simulink model "Control_linear2012b"  (R2012b)
settings: Solver=ode3  SolverMode=SingleTasking  StartTime=0.0  StopTime=50  FixedStep=0.005  RelTol=1e-3
values from neighbouring files (symbols this model uses):
  a1 = 0.2634    [int_for_newsimu.m]
  a2 = 1.6279    [int_for_newsimu.m]
  a3 = 25.6488    [int_for_newsimu.m]
  b1 = 0.531    [int_for_newsimu.m]
  b2 = 5.3292    [int_for_newsimu.m]
  epsilon_d = epsilon    (= 0)    [int_for_newsimu.m]
  fd = a3*cos(epsilon)*sin(theta)/b2    [int_for_newsimu.m]
  K_psi2theta = [1.8,0.2]    [int_for_newsimu.m]
  n = 0.9    [int_for_newsimu.m]
  theta_d = theta    (= 0)    [int_for_newsimu.m]
  w = 100    [int_for_newsimu.m]
undefined symbols (not defined in the file or in its folder): K
libraries: dspsrcs4 x9
settings Model: SimulationMode=external  ExtModeTrigDuration=200000  Creator=5420  LastModifiedBy=yk.L
settings DataIOCC: SignalLoggingSaveFormat=ModelDataLogs  SignalLoggingName=sigsOut
settings OptimizationCC: InitFltsAndDblsToZero=on
settings DebuggingCC: SaveWithParameterizedLinksMsg=none  SignalResolutionControl=TryResolveAllWithWarning  SolverPrmCheckMsg=none  MultiTaskDSMMsg=warning  MultiTaskCondExecSysMsg=none  FrameProcessingCompatibilityMsg=error
settings HardwareCC: ProdBitPerPointer=64  ProdLargestAtomicFloat=Float  ProdIntDivRoundTo=Zero  ProdEndianess=LittleEndian  ProdHWDeviceType=Specified
settings RTWCC: SystemTargetFile=rtwin.tlc  TemplateMakefile=rtwin.tmf  Description=Simulink Desktop Real-Time  ProcessScript=rtwin_make_rtw_hook  RTWCompilerOptimization=On
settings CodeAppCC: MaxIdLength=95
settings RTWinTargetCC: TargetPreCompLibLocation=D:\Program Files (x86)\MatlabR21019b\toolbox\sldrt\lib\win64  CodeReplacementLibrary=C89/C90 (ANSI)  ModelReferenceCompliant=off  CompOptLevelCompliant=off  RTWinDir=C:/PROGRA~1/MATLAB/R2012b/toolbox/rtw/targets/rtwin  TargetArch=win32  ExtModeMexFile=sldrtext

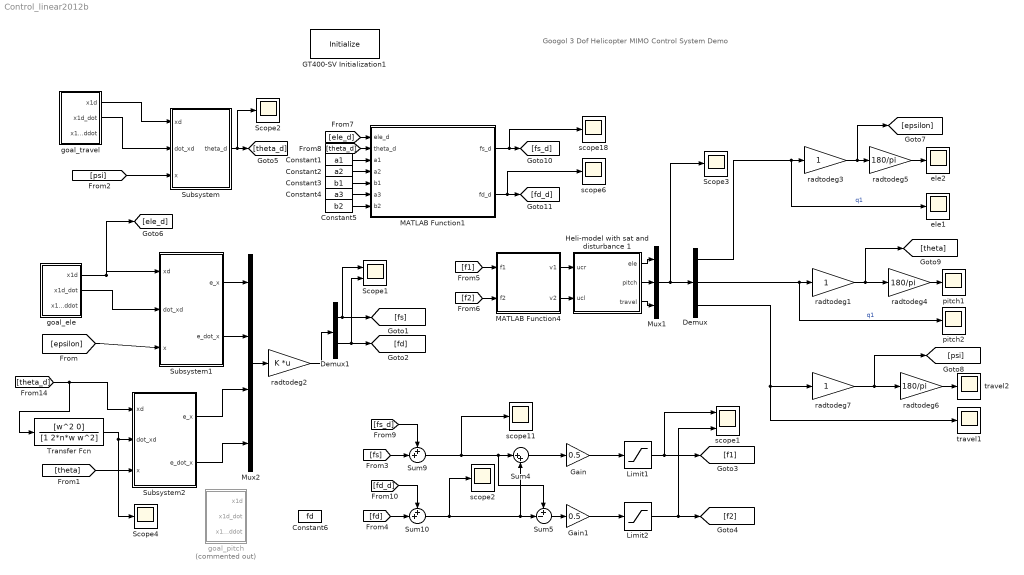
== system Control_linear2012b ==
  note: Googol 3 Dof Helicopter MIMO Control System Demo
  Constant1 : Constant  Value=a1
  Constant2 : Constant  Value=a2
  Constant3 : Constant  Value=b1
  Constant4 : Constant  Value=a3
  Constant5 : Constant  Value=b2
  Constant6 : Constant  Value=fd
  Demux : Demux  Outputs=3
  Demux1 : Demux  Outputs=2
  GT400-SV Initialization1 : S-Function  Priority=0  FunctionName=Initialize  Parameters=openloop  EnableBusSupport=off  mask(Initialize){openloop=1}
      mask prompts: openloop "Control loop:"
      mask help:
      | Initializing the googol GT400-SV motion control board.
      | Block parameter:
      |     Control loop:
      |          0: closed-loop control.
      |          1: opened-loop control.
      mask Help: This initialize block initializes the googol GT400-SV motion control board.
      mask Display: disp('Initialize \nGT400-SV');
  Gain : Gain  Gain=0.5
  Gain1 : Gain  Gain=0.5
  Heli-model with sat and disturbance 1 : Subsystem
  Limit1 : Saturate  UpperLimit=4  LowerLimit=0.05
  Limit2 : Saturate  UpperLimit=4  LowerLimit=0.05
  MATLAB Function1 : MATLAB Function  TreatAsAtomicUnit=on
  MATLAB Function4 : MATLAB Function  TreatAsAtomicUnit=on
  Mux1 : Mux  Inputs=3
  Mux2 : Mux
  Scope1 : Scope  NumInputPorts=2
      settings: YMin=-142.35203~-10.42115  YMax=297.12256~15.56883
  Scope2 : Scope
      settings: YMin=-0.02728  YMax=0.19696  SaveName=ScopeData2
  Scope3 : Scope
      settings: YMin=-1.59949  YMax=8.94541  SaveName=ScopeData18
  Scope4 : Scope
      settings: YMin=-0.02728  YMax=0.19696  SaveName=ScopeData6
  Subsystem : Subsystem
  Subsystem1 : Subsystem
  Subsystem2 : Subsystem
  Sum10 : Sum  Inputs=++|
  Sum4 : Sum  Inputs=|++
  Sum5 : Sum  Inputs=+-|
  Sum9 : Sum  Inputs=++|
  Transfer Fcn : TransferFcn  Numerator=[w^2 0]  Denominator=[1 2*n*w w^2]
  ele1 : Scope
      settings: YMin=-1.23857  YMax=0.24711  SaveName=elevation_real_data
  ele2 : Scope
      settings: YMin=4.45  YMax=4.775  SaveName=elevation_real_data1
  goal_ele : Subsystem
  goal_pitch : Subsystem  Commented=on
  goal_travel : Subsystem
  pitch1 : Scope
      settings: YMin=-12.5  YMax=-1  SaveName=pitch_real_data1
  pitch2 : Scope
      settings: YMin=-12.5  YMax=-1  SaveName=pitch_real_data
  radtodeg1 : Gain
  radtodeg2 : Gain  Gain=K  Multiplication=Matrix(K*u)
  radtodeg3 : Gain
  radtodeg4 : Gain  Gain=180/pi
  radtodeg5 : Gain  Gain=180/pi
  radtodeg6 : Gain  Gain=180/pi
  radtodeg7 : Gain
  scope1 : Scope  NumInputPorts=2
      settings: YMin=-0.44375~-0.44375  YMax=4.49375~4.49375  SaveName=ScopeData11
  scope{2,6,11,18} (4 alike) : Scope
      scope11 settings: YMin=-2.5  YMax=7.5  SaveName=fs_data
      scope18 settings: YMin=3.015  YMax=3.10151  SaveName=fs_d
      scope2 settings: YMin=-2.5  YMax=7.5  SaveName=fd_data
      scope6 settings: YMin=-0.2097  YMax=0.2097  SaveName=fd_d
  travel1 : Scope
      settings: YMin=295  YMax=327.5  SaveName=tralvel_real_data
  travel2 : Scope
      settings: YMin=295  YMax=327.5  SaveName=tralvel_real_data1
  wires:
  radtodeg5/1 -> ele2/1
  Demux/2 -> pitch2/1, radtodeg1/1  "q1"
  radtodeg6/1 -> travel2/1
  Demux/3 -> travel1/1, radtodeg7/1
  Mux1/1 -> Scope3/1, Demux/1
  Heli-model with sat and disturbance 1/1(ele) -> Mux1/1
  Heli-model with sat and disturbance 1/2(pitch) -> Mux1/2
  Heli-model with sat and disturbance 1/3(travel) -> Mux1/3
  Demux/1 -> ele1/1, radtodeg3/1  "q1"
  radtodeg4/1 -> pitch1/1
  Mux2/1 -> radtodeg2/1
  radtodeg2/1 -> Demux1/1
  Sum10/1 -> scope2/1, Sum5/2, Sum4/2
  Sum4/1 -> Gain/1
  Sum9/1 -> scope11/1, Sum5/1, Sum4/1
  Sum5/1 -> Gain1/1
  Gain/1 -> Limit1/1
  Gain1/1 -> Limit2/1
  Limit1/1 -> scope1/1, [f1]
  Limit2/1 -> [f2], scope1/2
  Demux1/1 -> Scope1/1, [fs]
  Demux1/2 -> Scope1/2, [fd]
  [f1] -> MATLAB Function4/1(f1)
  [f2] -> MATLAB Function4/2(f2)
  radtodeg1/1 -> [theta], radtodeg4/1
  radtodeg3/1 -> [epsilon], radtodeg5/1
  radtodeg7/1 -> radtodeg6/1, [psi]
  [theta_d] -> Transfer Fcn/1, Subsystem2/1(xd)
  [fs] -> Sum9/2
  [fd] -> Sum10/2
  [ele_d] -> MATLAB Function1/1(ele_d)
  [theta_d] -> MATLAB Function1/2(theta_d)
  Constant1/1 -> MATLAB Function1/3(a1)
  Constant2/1 -> MATLAB Function1/4(a2)
  Constant3/1 -> MATLAB Function1/5(b1)
  Constant4/1 -> MATLAB Function1/6(a3)
  Constant5/1 -> MATLAB Function1/7(b2)
  MATLAB Function1/1(fs_d) -> scope18/1, [fs_d]
  MATLAB Function1/2(fd_d) -> scope6/1, [fd_d]
  goal_travel/1(x1d) -> Subsystem/1(xd)
  goal_travel/2(x1d_dot) -> Subsystem/2(dot_xd)
  [psi] -> Subsystem/3(x)
  goal_ele/1(x1d) -> [ele_d], Subsystem1/1(xd)
  goal_ele/2(x1d_dot) -> Subsystem1/2(dot_xd)
  [epsilon] -> Subsystem1/3(x)
  Transfer Fcn/1 -> Subsystem2/2(dot_xd), Scope4/1
  [theta] -> Subsystem2/3(x)
  [fs_d] -> Sum9/1
  [fd_d] -> Sum10/1
  Subsystem1/1(e_x) -> Mux2/1
  Subsystem1/2(e_dot_x) -> Mux2/2
  Subsystem2/1(e_x) -> Mux2/3
  Subsystem2/2(e_dot_x) -> Mux2/4
  Subsystem/1(theta_d) -> Scope2/1, [theta_d]
  MATLAB Function4/1(v1) -> Heli-model with sat and disturbance 1/1(ucr)
  MATLAB Function4/2(v2) -> Heli-model with sat and disturbance 1/2(ucl)

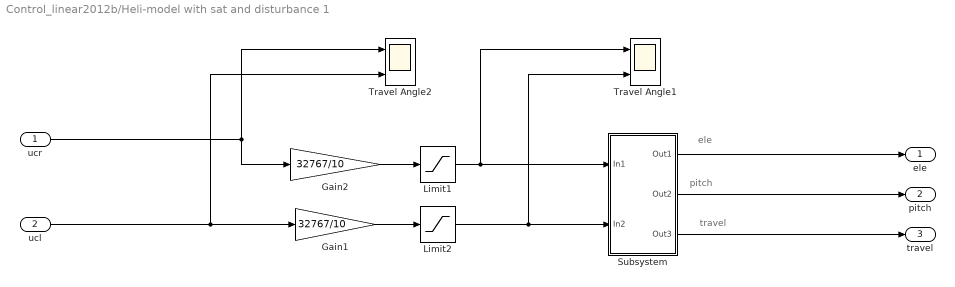
== system Control_linear2012b/Heli-model with sat and disturbance 1 ==
  note: travel
  note: pitch
  note: ele
  ucr : Inport
  ucl : Inport  Port=2
  Gain1 : Gain  Gain=32767/10
  Gain2 : Gain  Gain=32767/10
  Limit1 : Saturate  UpperLimit=15000  LowerLimit=-15000
  Limit2 : Saturate  UpperLimit=15000  LowerLimit=-15000
  Subsystem : Subsystem
  Travel Angle1 : Scope  NumInputPorts=2
      settings: TimeRange=200  YMin=0~0  YMax=3500~3500  SaveName=travel1  MaxDataPoints=200000
  Travel Angle2 : Scope  NumInputPorts=2
      settings: TimeRange=200  YMin=0.3~0.3  YMax=0.7~0.7  SaveName=travel  MaxDataPoints=200000
  ele : Outport
  pitch : Outport  Port=2
  travel : Outport  Port=3
  wires:
  Subsystem/1(Out1) -> ele/1
  Subsystem/2(Out2) -> pitch/1
  Subsystem/3(Out3) -> travel/1
  Gain2/1 -> Limit1/1
  Gain1/1 -> Limit2/1
  Limit1/1 -> Travel Angle1/1, Subsystem/1(In1)
  Limit2/1 -> Travel Angle1/2, Subsystem/2(In2)
  ucr/1 -> Gain2/1, Travel Angle2/1
  ucl/1 -> Travel Angle2/2, Gain1/1

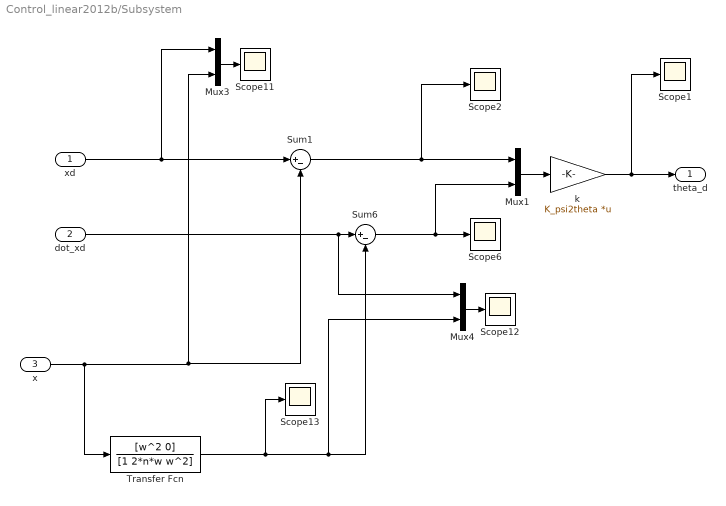
== system Control_linear2012b/Subsystem ==
  xd : Inport
  dot_xd : Inport  Port=2
  x : Inport  Port=3
  Mux1 : Mux  Inputs=2
  Mux3 : Mux  Inputs=2
  Mux4 : Mux  Inputs=2
  Scope{1..2,6,11..13} (6 alike) : Scope
      Scope1 settings: YMin=-0.02728  YMax=0.19696
      Scope11 settings: TimeRange=50  YMin=-0.02184  YMax=0.19654  SaveName=ScopeData3
      Scope12 settings: YMin=-0.49275  YMax=-0.4885  SaveName=ScopeData16
      Scope13 settings: YMin=0.0013  YMax=0.0027  SaveName=ScopeData17
      Scope2 settings: YMin=-0.02201  YMax=0.19637  SaveName=ScopeData19
      Scope6 settings: YMin=-0.0879  YMax=0.00986  SaveName=ScopeData20
  Sum1 : Sum  Inputs=|+-
  Sum6 : Sum  Inputs=|+-
  Transfer Fcn : TransferFcn  Numerator=[w^2 0]  Denominator=[1 2*n*w w^2]
  k : Gain  Gain=K_psi2theta  Multiplication=Matrix(K*u)
  theta_d : Outport
  wires:
  dot_xd/1 -> Mux4/1, Sum6/1
  x/1 -> Transfer Fcn/1, Sum1/2, Mux3/2
  Transfer Fcn/1 -> Scope13/1, Mux4/2, Sum6/2
  Sum6/1 -> Mux1/2, Scope6/1
  Mux3/1 -> Scope11/1
  Mux4/1 -> Scope12/1
  Sum1/1 -> Mux1/1, Scope2/1
  xd/1 -> Mux3/1, Sum1/1
  Mux1/1 -> k/1
  k/1 -> Scope1/1, theta_d/1

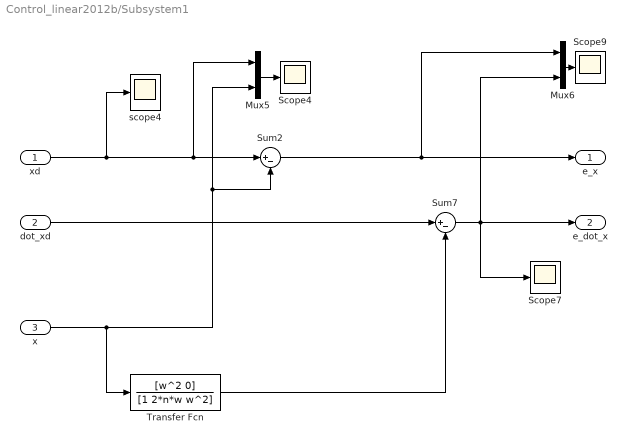
== system Control_linear2012b/Subsystem1 ==
  xd : Inport
  dot_xd : Inport  Port=2
  x : Inport  Port=3
  Mux5 : Mux  Inputs=2
  Mux6 : Mux  Inputs=2
  Scope4 : Scope
      settings: YMin=-0.61494  YMax=0.08442  SaveName=ScopeData4
  Scope7 : Scope
      settings: YMin=-1  YMax=12  SaveName=ScopeData7
  Scope9 : Scope
      settings: YMin=-0.52  YMax=-0.4875  SaveName=ScopeData12
  Sum2 : Sum  Inputs=|+-
  Sum7 : Sum  Inputs=|+-
  Transfer Fcn : TransferFcn  Numerator=[w^2 0]  Denominator=[1 2*n*w w^2]
  scope4 : Scope
      settings: YMin=-2.5  YMax=7.5  SaveName=ele_d_data  DataFormat=Structure
  e_x : Outport
  e_dot_x : Outport  Port=2
  wires:
  xd/1 -> Mux5/1, Sum2/1, scope4/1
  Mux6/1 -> Scope9/1
  Mux5/1 -> Scope4/1
  Transfer Fcn/1 -> Sum7/2
  x/1 -> Transfer Fcn/1, Mux5/2, Sum2/2
  Sum7/1 -> Mux6/2, e_dot_x/1, Scope7/1
  Sum2/1 -> e_x/1, Mux6/1
  dot_xd/1 -> Sum7/1

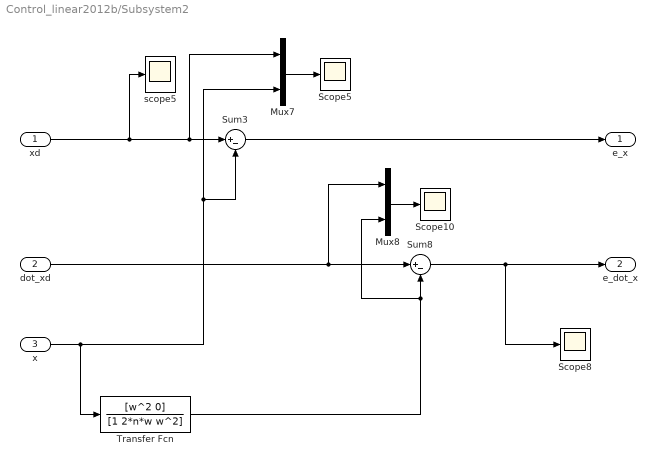
== system Control_linear2012b/Subsystem2 ==
  xd : Inport
  dot_xd : Inport  Port=2
  x : Inport  Port=3
  Mux7 : Mux  Inputs=2
  Mux8 : Mux  Inputs=2
  Scope10 : Scope
      settings: YMin=-0.08392  YMax=0.52488  SaveName=ScopeData13
  Scope5 : Scope
      settings: YMin=-0.02741  YMax=0.19697  SaveName=ScopeData5
  Scope8 : Scope
      settings: YMin=-1  YMax=12  SaveName=ScopeData10
  Sum3 : Sum  Inputs=|+-
  Sum8 : Sum  Inputs=|+-
  Transfer Fcn : TransferFcn  Numerator=[w^2 0]  Denominator=[1 2*n*w w^2]
  scope5 : Scope
      settings: YMin=-2.5  YMax=7.5  SaveName=pitch_d_data  DataFormat=Structure
  e_x : Outport
  e_dot_x : Outport  Port=2
  wires:
  Sum3/1 -> e_x/1
  Transfer Fcn/1 -> Sum8/2, Mux8/2
  Sum8/1 -> Scope8/1, e_dot_x/1
  xd/1 -> scope5/1, Mux7/1, Sum3/1
  x/1 -> Transfer Fcn/1, Sum3/2, Mux7/2
  Mux8/1 -> Scope10/1
  dot_xd/1 -> Sum8/1, Mux8/1
  Mux7/1 -> Scope5/1

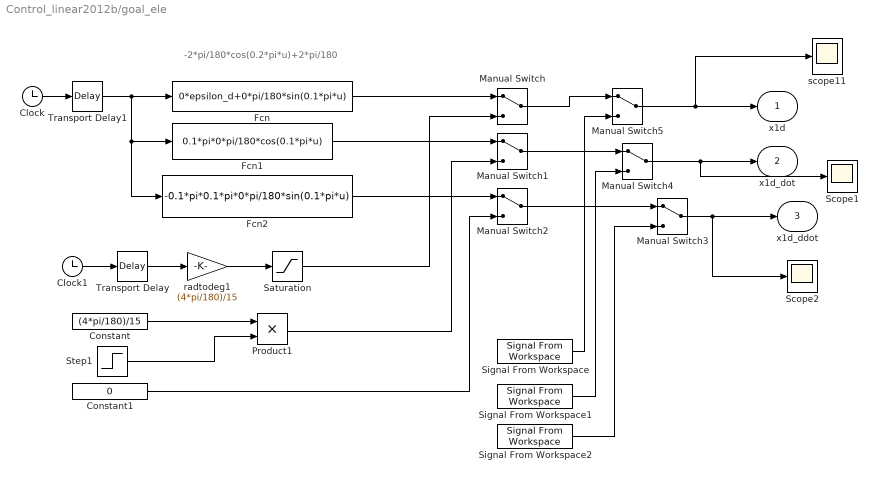
== system Control_linear2012b/goal_ele ==
  note: -2*pi/180*cos(0.2*pi*u)+2*pi/180
  Clock : Clock
  Clock1 : Clock
  Constant : Constant  Value=(4*pi/180)/15
  Constant1 : Constant  Value=0
  Fcn : Fcn  Expr=0*epsilon_d+0*pi/180*sin(0.1*pi*u)
  Fcn1 : Fcn  Expr=0.1*pi*0*pi/180*cos(0.1*pi*u)
  Fcn2 : Fcn  Expr=-0.1*pi*0.1*pi*0*pi/180*sin(0.1*pi*u)
  Manual Switch{,1..5} (6 alike) : ManualSwitch
  Product1 : Product  RndMeth=Zero
  Saturation : Saturate  UpperLimit=(4*pi/180)  LowerLimit=-(4*pi/180)
  Scope1 : Scope
      settings: YMin=-10  YMax=10  SaveName=ScopeData8
  Scope2 : Scope
      settings: YMin=-10  YMax=10  SaveName=ScopeData9
  Signal From Workspace : dspsrcs4/Signal From Workspace  X=epsilon  Ts=0.005  nsamps=1  OutputAfterFinalValue=Setting to zero  ignoreOrWarnInputAndFrameLengths=off
  Signal From Workspace1 : dspsrcs4/Signal From Workspace  X=dot_epsilon  Ts=0.005  nsamps=1  OutputAfterFinalValue=Setting to zero  ignoreOrWarnInputAndFrameLengths=off
  Signal From Workspace2 : dspsrcs4/Signal From Workspace  X=ddot_epsilon  Ts=0.005  nsamps=1  OutputAfterFinalValue=Setting to zero  ignoreOrWarnInputAndFrameLengths=off
  Step1 : Step  Time=12  SampleTime=0
  Transport Delay : TransportDelay  DelayTime=12
  Transport Delay1 : TransportDelay  DelayTime=0
  radtodeg1 : Gain  Gain=(4*pi/180)/15
  scope11 : Scope
      settings: YMin=-2.5  YMax=7.5  SaveName=ele_d_data
  x1d : Outport
  x1d_dot : Outport  Port=2
  x1d_ddot : Outport  Port=3
  wires:
  Clock/1 -> Transport Delay1/1
  Clock1/1 -> Transport Delay/1
  Transport Delay/1 -> radtodeg1/1
  radtodeg1/1 -> Saturation/1
  Fcn/1 -> Manual Switch/1
  Fcn1/1 -> Manual Switch1/1
  Fcn2/1 -> Manual Switch2/1
  Manual Switch2/1 -> Manual Switch3/1
  Saturation/1 -> Manual Switch/2
  Constant1/1 -> Manual Switch2/2
  Constant/1 -> Product1/1
  Step1/1 -> Product1/2
  Product1/1 -> Manual Switch1/2
  Transport Delay1/1 -> Fcn1/1, Fcn2/1, Fcn/1
  Signal From Workspace2/1 -> Manual Switch3/2
  Manual Switch3/1 -> Scope2/1, x1d_ddot/1
  Signal From Workspace1/1 -> Manual Switch4/2
  Manual Switch1/1 -> Manual Switch4/1
  Manual Switch4/1 -> Scope1/1, x1d_dot/1
  Manual Switch/1 -> Manual Switch5/1
  Signal From Workspace/1 -> Manual Switch5/2
  Manual Switch5/1 -> scope11/1, x1d/1

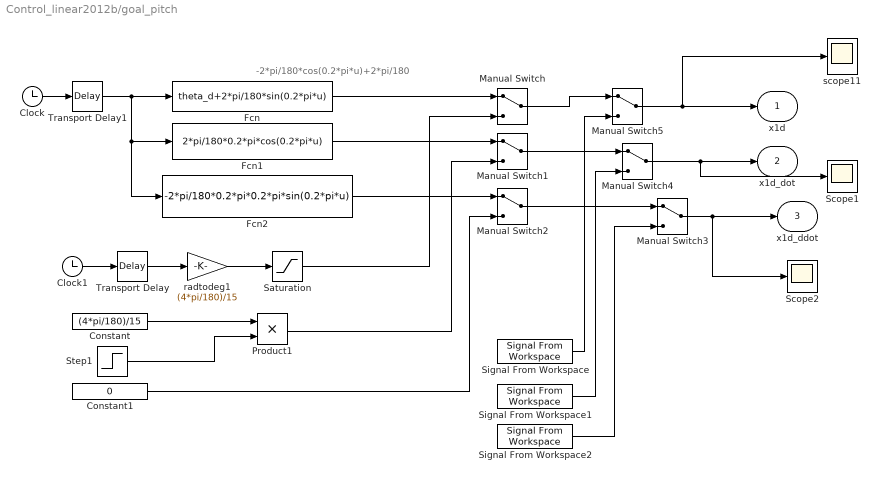
== system Control_linear2012b/goal_pitch ==
  note: -2*pi/180*cos(0.2*pi*u)+2*pi/180
  Clock : Clock
  Clock1 : Clock
  Constant : Constant  Value=(4*pi/180)/15
  Constant1 : Constant  Value=0
  Fcn : Fcn  Expr=theta_d+2*pi/180*sin(0.2*pi*u)
  Fcn1 : Fcn  Expr=2*pi/180*0.2*pi*cos(0.2*pi*u)
  Fcn2 : Fcn  Expr=-2*pi/180*0.2*pi*0.2*pi*sin(0.2*pi*u)
  Manual Switch{,1..5} (6 alike) : ManualSwitch
  Product1 : Product  RndMeth=Zero
  Saturation : Saturate  UpperLimit=(4*pi/180)  LowerLimit=-(4*pi/180)
  Scope1 : Scope
      settings: YMin=-10  YMax=10  SaveName=ScopeData8
  Scope2 : Scope
      settings: YMin=-10  YMax=10  SaveName=ScopeData9
  Signal From Workspace : dspsrcs4/Signal From Workspace  X=epsilon  Ts=0.005  nsamps=1  OutputAfterFinalValue=Setting to zero  ignoreOrWarnInputAndFrameLengths=off
  Signal From Workspace1 : dspsrcs4/Signal From Workspace  X=dot_epsilon  Ts=0.005  nsamps=1  OutputAfterFinalValue=Setting to zero  ignoreOrWarnInputAndFrameLengths=off
  Signal From Workspace2 : dspsrcs4/Signal From Workspace  X=ddot_epsilon  Ts=0.005  nsamps=1  OutputAfterFinalValue=Setting to zero  ignoreOrWarnInputAndFrameLengths=off
  Step1 : Step  Time=12  SampleTime=0
  Transport Delay : TransportDelay  DelayTime=12
  Transport Delay1 : TransportDelay  DelayTime=0
  radtodeg1 : Gain  Gain=(4*pi/180)/15
  scope11 : Scope
      settings: YMin=-2.5  YMax=7.5  SaveName=pitch_d_data
  x1d : Outport
  x1d_dot : Outport  Port=2
  x1d_ddot : Outport  Port=3
  wires:
  Clock/1 -> Transport Delay1/1
  Clock1/1 -> Transport Delay/1
  Transport Delay/1 -> radtodeg1/1
  radtodeg1/1 -> Saturation/1
  Fcn/1 -> Manual Switch/1
  Fcn1/1 -> Manual Switch1/1
  Fcn2/1 -> Manual Switch2/1
  Manual Switch2/1 -> Manual Switch3/1
  Saturation/1 -> Manual Switch/2
  Constant1/1 -> Manual Switch2/2
  Constant/1 -> Product1/1
  Step1/1 -> Product1/2
  Product1/1 -> Manual Switch1/2
  Transport Delay1/1 -> Fcn1/1, Fcn2/1, Fcn/1
  Signal From Workspace2/1 -> Manual Switch3/2
  Manual Switch3/1 -> Scope2/1, x1d_ddot/1
  Signal From Workspace1/1 -> Manual Switch4/2
  Manual Switch1/1 -> Manual Switch4/1
  Manual Switch4/1 -> Scope1/1, x1d_dot/1
  Manual Switch/1 -> Manual Switch5/1
  Signal From Workspace/1 -> Manual Switch5/2
  Manual Switch5/1 -> scope11/1, x1d/1

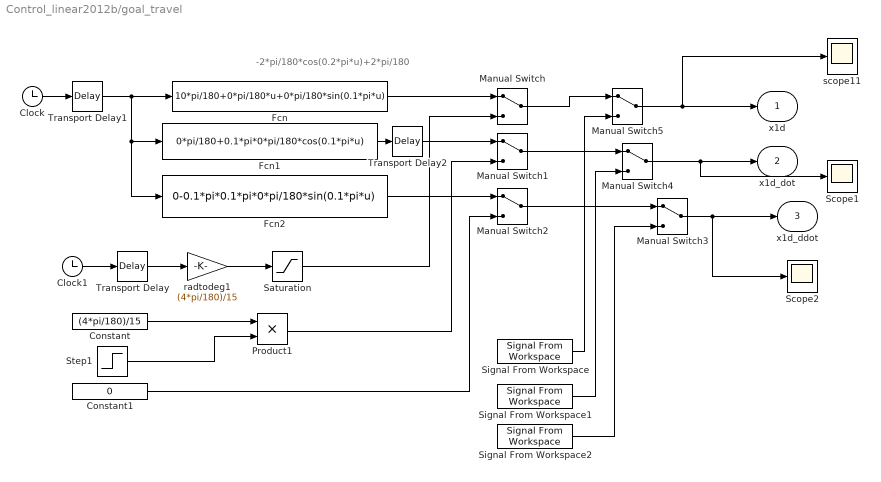
== system Control_linear2012b/goal_travel ==
  note: -2*pi/180*cos(0.2*pi*u)+2*pi/180
  Clock : Clock
  Clock1 : Clock
  Constant : Constant  Value=(4*pi/180)/15
  Constant1 : Constant  Value=0
  Fcn : Fcn  Expr=10*pi/180+0*pi/180*u+0*pi/180*sin(0.1*pi*u)
  Fcn1 : Fcn  Expr=0*pi/180+0.1*pi*0*pi/180*cos(0.1*pi*u)
  Fcn2 : Fcn  Expr=0-0.1*pi*0.1*pi*0*pi/180*sin(0.1*pi*u)
  Manual Switch{,1..5} (6 alike) : ManualSwitch
  Product1 : Product  RndMeth=Zero
  Saturation : Saturate  UpperLimit=(4*pi/180)  LowerLimit=-(4*pi/180)
  Scope1 : Scope
      settings: YMin=-0.01309  YMax=0.11781  SaveName=ScopeData8
  Scope2 : Scope
      settings: YMin=-1.00000  YMax=1.00000  SaveName=ScopeData9
  Signal From Workspace : dspsrcs4/Signal From Workspace  X=epsilon  Ts=0.005  nsamps=1  OutputAfterFinalValue=Setting to zero  ignoreOrWarnInputAndFrameLengths=off
  Signal From Workspace1 : dspsrcs4/Signal From Workspace  X=dot_epsilon  Ts=0.005  nsamps=1  OutputAfterFinalValue=Setting to zero  ignoreOrWarnInputAndFrameLengths=off
  Signal From Workspace2 : dspsrcs4/Signal From Workspace  X=ddot_epsilon  Ts=0.005  nsamps=1  OutputAfterFinalValue=Setting to zero  ignoreOrWarnInputAndFrameLengths=off
  Step1 : Step  Time=12  SampleTime=0
  Transport Delay : TransportDelay  DelayTime=12
  Transport Delay1 : TransportDelay  DelayTime=10
  Transport Delay2 : TransportDelay  DelayTime=10
  radtodeg1 : Gain  Gain=(4*pi/180)/15
  scope11 : Scope
      settings: YMin=-2.5  YMax=7.5  SaveName=travel_d_data
  x1d : Outport
  x1d_dot : Outport  Port=2
  x1d_ddot : Outport  Port=3
  wires:
  Clock/1 -> Transport Delay1/1
  Clock1/1 -> Transport Delay/1
  Transport Delay/1 -> radtodeg1/1
  radtodeg1/1 -> Saturation/1
  Manual Switch2/1 -> Manual Switch3/1
  Saturation/1 -> Manual Switch/2
  Constant1/1 -> Manual Switch2/2
  Constant/1 -> Product1/1
  Step1/1 -> Product1/2
  Product1/1 -> Manual Switch1/2
  Transport Delay1/1 -> Fcn1/1, Fcn2/1, Fcn/1
  Signal From Workspace2/1 -> Manual Switch3/2
  Manual Switch3/1 -> Scope2/1, x1d_ddot/1
  Signal From Workspace1/1 -> Manual Switch4/2
  Manual Switch1/1 -> Manual Switch4/1
  Manual Switch4/1 -> Scope1/1, x1d_dot/1
  Manual Switch/1 -> Manual Switch5/1
  Signal From Workspace/1 -> Manual Switch5/2
  Manual Switch5/1 -> scope11/1, x1d/1
  Fcn/1 -> Manual Switch/1
  Fcn1/1 -> Transport Delay2/1
  Fcn2/1 -> Manual Switch2/1
  Transport Delay2/1 -> Manual Switch1/1

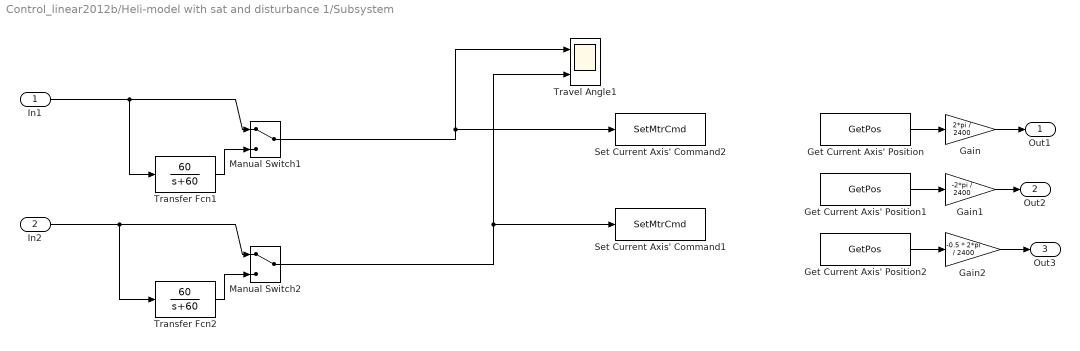
== system Control_linear2012b/Heli-model with sat and disturbance 1/Subsystem ==
  In1 : Inport
  In2 : Inport  Port=2
  Gain : Gain  Gain=2*pi / 2400  SaturateOnIntegerOverflow=on  OutDataTypeStr=Inherit: Same as input  ParamDataTypeStr=Inherit: Same as input
  Gain1 : Gain  Gain=-2*pi / 2400  SaturateOnIntegerOverflow=on  OutDataTypeStr=Inherit: Same as input  ParamDataTypeStr=Inherit: Same as input
  Gain2 : Gain  Gain=-0.5 * 2*pi / 2400  SaturateOnIntegerOverflow=on  OutDataTypeStr=Inherit: Same as input  ParamDataTypeStr=Inherit: Same as input
  Get Current Axis' Position : S-Function  Priority=1  FunctionName=GetPos  Parameters=axis  EnableBusSupport=off  mask(GetPos){axis=2}
      mask prompts: axis "Axis number:"
      mask help:
      | Getting the current axis position value in encoder' counts.
      | Block parameter:
      |     Axis number:  must be between 1 and 6, default is 1.
      | Block output:
      |     1~4: current axis' encoder reading counts.
      |     5/6: assistant encoder 1/2 reading counts.
      mask Help:
      | This block, GetPos, is intended for getting the current axis position value in encoder' counts. This value represents the actual position for the axis
      | at the current sample time. This command operates for all profile modes.
      | The value returned is a 32-bit signed number with units of counts.
      | The range is -1,073,741,824 to 1,073,741,823.
      | 
      | You can recalculate obtained value into meter units via multiplication by the scaler coefficient .
      | 
      | Block parameter:
      |     Axis number:  must be between 1 and 4, default is 1.
      | Block input: none.
      | Block output:
      |         1~4: current axis' encoder reading counts.
      |         5/6: assistant encoder 1/2 reading counts.
      mask Display:
      | disp('GetPos');
      | port_label('output', 1, 'Pos');
  Get Current Axis' Position1 : S-Function  Priority=1  FunctionName=GetPos  Parameters=axis  EnableBusSupport=off  mask(GetPos){axis=1}
      mask prompts: axis "Axis number:"
      mask help:
      | Getting the current axis position value in encoder' counts.
      | Block parameter:
      |     Axis number:  must be between 1 and 6, default is 1.
      | Block output:
      |     1~4: current axis' encoder reading counts.
      |     5/6: assistant encoder 1/2 reading counts.
      mask Help:
      | This block, GetPos, is intended for getting the current axis position value in encoder' counts. This value represents the actual position for the axis
      | at the current sample time. This command operates for all profile modes.
      | The value returned is a 32-bit signed number with units of counts.
      | The range is -1,073,741,824 to 1,073,741,823.
      | 
      | You can recalculate obtained value into meter units via multiplication by the scaler coefficient .
      | 
      | Block parameter:
      |     Axis number:  must be between 1 and 4, default is 1.
      | Block input: none.
      | Block output:
      |         1~4: current axis' encoder reading counts.
      |         5/6: assistant encoder 1/2 reading counts.
      mask Display:
      | disp('GetPos');
      | port_label('output', 1, 'Pos');
  Get Current Axis' Position2 : S-Function  Priority=1  FunctionName=GetPos  Parameters=axis  EnableBusSupport=off  mask(GetPos){axis=3}
      mask prompts: axis "Axis number:"
      mask help:
      | Getting the current axis position value in encoder' counts.
      | Block parameter:
      |     Axis number:  must be between 1 and 6, default is 1.
      | Block output:
      |     1~4: current axis' encoder reading counts.
      |     5/6: assistant encoder 1/2 reading counts.
      mask Help:
      | This block, GetPos, is intended for getting the current axis position value in encoder' counts. This value represents the actual position for the axis
      | at the current sample time. This command operates for all profile modes.
      | The value returned is a 32-bit signed number with units of counts.
      | The range is -1,073,741,824 to 1,073,741,823.
      | 
      | You can recalculate obtained value into meter units via multiplication by the scaler coefficient .
      | 
      | Block parameter:
      |     Axis number:  must be between 1 and 4, default is 1.
      | Block input: none.
      | Block output:
      |         1~4: current axis' encoder reading counts.
      |         5/6: assistant encoder 1/2 reading counts.
      mask Display:
      | disp('GetPos');
      | port_label('output', 1, 'Pos');
  Manual Switch1 : ManualSwitch
  Manual Switch2 : ManualSwitch
  Set Current Axis' Command1 : S-Function  Priority=1  FunctionName=SetMtrCmd  Parameters=axis  EnableBusSupport=off  mask(SetMtrCmd){axis=1}
      mask prompts: axis "Axis number:"
      mask help:
      | Settting the current axis' voltage.
      | Block parameter:
      |     Axis number:  must be between 1 and 4, default is 1.
      | Block input:
      |     the current axis' voltage.
      mask Help:
      | This SetMtrCmd settting the current axis' voltage.
      | Block parameter:
      |     Axis number:  must be between 1 and 4, default is 1.
      mask Display:
      | disp('          SetMtrCmd');
      | port_label('input', 1, 'Vol');
  Set Current Axis' Command2 : S-Function  Priority=1  FunctionName=SetMtrCmd  Parameters=axis  EnableBusSupport=off  mask(SetMtrCmd){axis=2}
      mask prompts: axis "Axis number:"
      mask help:
      | Settting the current axis' voltage.
      | Block parameter:
      |     Axis number:  must be between 1 and 4, default is 1.
      | Block input:
      |     the current axis' voltage.
      mask Help:
      | This SetMtrCmd settting the current axis' voltage.
      | Block parameter:
      |     Axis number:  must be between 1 and 4, default is 1.
      mask Display:
      | disp('          SetMtrCmd');
      | port_label('input', 1, 'Vol');
  Transfer Fcn1 : TransferFcn  Numerator=[60]  Denominator=[1 60]
  Transfer Fcn2 : TransferFcn  Numerator=[60]  Denominator=[1 60]
  Travel Angle1 : Scope  NumInputPorts=2
      settings: TimeRange=200  YMin=1000~1250  YMax=2300~1950  SaveName=travel4  MaxDataPoints=200000
  Out1 : Outport
  Out2 : Outport  Port=2
  Out3 : Outport  Port=3
  wires:
  Get Current Axis' Position/1 -> Gain/1
  Get Current Axis' Position1/1 -> Gain1/1
  Get Current Axis' Position2/1 -> Gain2/1
  Gain/1 -> Out1/1
  Gain1/1 -> Out2/1
  Gain2/1 -> Out3/1
  Manual Switch1/1 -> Travel Angle1/1, Set Current Axis' Command2/1
  Manual Switch2/1 -> Travel Angle1/2, Set Current Axis' Command1/1
  In1/1 -> Transfer Fcn1/1, Manual Switch1/1
  Transfer Fcn1/1 -> Manual Switch1/2
  In2/1 -> Transfer Fcn2/1, Manual Switch2/1
  Transfer Fcn2/1 -> Manual Switch2/2

== matlab function Control_linear2012b/MATLAB Function1 ==
  data: fs_d output; ele_d input; fd_d output; theta_d input; a1 input; a2 input; b1 input; a3 input; b2 input
function [fs_d,fd_d] = fcn(ele_d,theta_d,a1,a2,b1,a3,b2)
theta = theta_d;
epsilon = ele_d;

fs_d = (a1*cos(theta)*sin(epsilon)+a2*cos(epsilon))/(b1*cos(theta));
fd_d = a3*cos(epsilon)*sin(theta)/b2;

== matlab function Control_linear2012b/MATLAB Function4 ==
  data: f1 input; v1 output; f2 input; v2 output
function [v1,v2] = fcn(f1,f2)

v1= 1.677*f1^0.4716 - 0.3538;
v2= 1.677*f2^0.4716 - 0.3538;
